simulink model "ava4"  (R2017b)
settings: Solver=VariableStepAuto  StartTime=0.0  StopTime=10.0  RelTol=1e-3
settings Model: Creator=hbourbou  LastModifiedBy=hbourbou

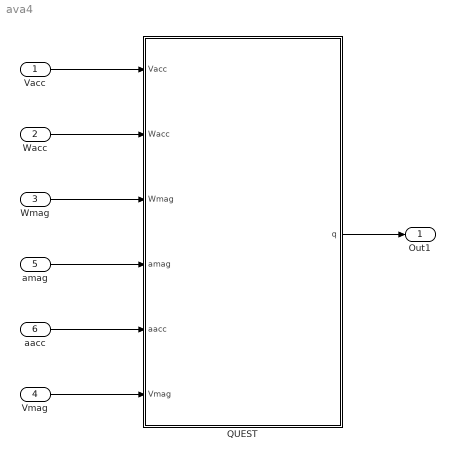
== system ava4 ==
  Vacc : Inport  PortDimensions=3
  Wacc : Inport  Port=2  PortDimensions=3
  Wmag : Inport  Port=3  PortDimensions=3
  Vmag : Inport  Port=4  PortDimensions=3
  amag : Inport  Port=5
  aacc : Inport  Port=6
  QUEST : MATLAB Function  TreatAsAtomicUnit=on
  Out1 : Outport
  wires:
  Vacc/1 -> QUEST/1(Vacc)
  Wacc/1 -> QUEST/2(Wacc)
  Wmag/1 -> QUEST/3(Wmag)
  Vmag/1 -> QUEST/6(Vmag)
  amag/1 -> QUEST/4(amag)
  aacc/1 -> QUEST/5(aacc)
  QUEST/1(q) -> Out1/1

== matlab function ava4/QUEST ==
  data: Vacc input double; Wacc input double; Wmag input double; q output double; amag input double; aacc input double; Vmag input double
function q=QUEST(Vacc,Wacc,Wmag,amag,aacc,Vmag)
%#codegen

% Quaternion Estimator (QUEST)
% Vivek Nagabhushan, Millenium Engineering and Integration Company
% 05/24/2013
% References:
% 1. Shuster, M. D. and Oh, S. D., 'Three Axis Attitude Determination from
% Vector Observations', Journal of Guidance and Control, Vol. 4,
% No. 1, pp. 70-77, 1981
% 2. Markley, F. L. and Mortari, D., "Quaternion Attitude Estimation Using
% Vector Observations" Journal of the Astronautical Sciences, Vol. 48,
% No.2, pp. 359-380, 2000

% Inputs
% 1. Wgps is a 3 X n matrix where jth column of Wgps is the jth unit vector
%    observation in the body coordinate basis derived from known positions
%    of GPS sensors
%    Wmag and Wdmag are similarly defined and obtained using magnetic field measurement and Bdot
%    (derivative of magnetometer measurements),respectively.

% 2. Vgps is a 3 X n matrix where jth column of Vgps is the jth unit vector
%    observation in the reference (ECF) coordinate basis derived from GPS measurements
%    Vmag and Vdmag are similarly defined and obtained using the
%    knowledgede of the sensor position and WMM.

% 3. agps is a 1 X n matrix where the jth term is the weighting on the jth set
% of vector observations obtained using GPS measurements

% Output
% 1. The optimal quaternion that represents the transfomation from the body
% coordinate basis to the inertial coordinate basis

W=[Wmag Wacc];
V=[Vmag Vacc];
A=[amag aacc];

rows=size(W,2);

B=zeros(3,3);

for j=1:rows
    B=B+A(j)*(W(1:3,j)*V(1:3,j)');
end

sigma=B(1,1)+B(2,2)+B(3,3); % Trace of B

z=[B(2,3)-B(3,2) ; B(3,1)-B(1,3) ; B(1,2)-B(2,1)];

S=B+B';

adjS=[S(2,2)*S(3,3)-S(2,3)*S(3,2) S(1,3)*S(3,2)-S(1,2)*S(3,3) S(1,2)*S(2,3)-S(1,3)*S(2,2); % Adjugate of S
      S(2,3)*S(3,1)-S(2,1)*S(3,3) S(1,1)*S(3,3)-S(1,3)*S(3,1) S(2,1)*S(1,3)-S(1,1)*S(2,3);
      S(2,1)*S(3,2)-S(2,2)*S(3,1) S(1,2)*S(3,1)-S(1,1)*S(3,2) S(1,1)*S(2,2)-S(1,2)*S(2,1)];

kappa=adjS(1,1)+adjS(2,2)+adjS(3,3); %Trace of adjS

Delta=S(1,1)*adjS(1,1)+S(1,2)*adjS(1,2)+S(1,3)*adjS(1,3); % Determinant of S

a=sigma^2-kappa;
b=sigma^2+z'*z;
c=Delta+z'*S*z;
d=z'*(S^2)*z;

l=a+b;
m=c;
n=a*b+c*sigma-d;

lambda=1;
epsilon=1;

while epsilon>=0.00001 || epsilon<=-0.00001 % Newton-Raphson method for determining lambda (which is close to 1)
    ce=lambda^4-l*lambda^2-m*lambda+n;
    dce=4*lambda^3-2*l*lambda-m;
lambda= lambda-((ce)/(dce));
epsilon=lambda^4-l*lambda^2-m*lambda+n;
end

alpha=lambda^2-sigma^2+kappa;
beta=lambda-sigma;
gamma=(lambda+sigma)*alpha-Delta;

x=(alpha*eye(3)+beta*S+S^2)*z;

q=[x;gamma]/(sqrt(gamma^2+x'*x));

% Note: The quest method presents a singularity at a 180 degree rotation or
% when the fourth component of the quaternion is zero. With a good orbit
% inclination, it is unlikely that the orientation of the vehicle would
% have a 180 degree quaternion angle. If in case, this occurs, we can
% implement pseudo rotations [Shuster (1981)] or implement SVD method
% [Markely and Mortari 2000] as an intermediate step.
